simulink model "solar_thermal_sym"  (R2024b)
settings: Solver=FixedStepAuto  StartTime=0.0  StopTime=24*3600  FixedStep=60  RelTol=1e-3
values from neighbouring files (symbols this model uses):
  FR_consumption = 0*min    [Consumption_profiles.m]
  I_sym = I_feb    [Consumption_profiles.m]
  T_mains = 12    [Consumption_profiles.m]
  Ta_sym = Ta_feb    [Consumption_profiles.m]
  TR_consumption = 0*min    [Consumption_profiles.m]
undefined symbols (not defined in the file or in its folder): A, c, epsilon, eta_0, m_c, M_s, T_home, tank_LC, Tin_0, Ts_0, U
settings Model: Creator=edoardomurgia  LastModifiedBy=edoardomurgia
settings DataIOCC: ReturnWorkspaceOutputs=off
settings DebuggingCC: AlgebraicLoopMsg=none

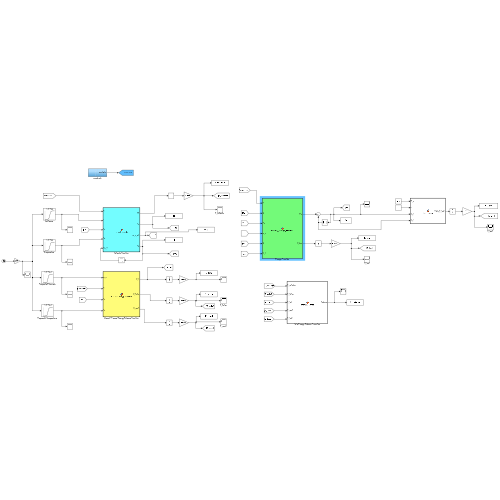
[thumbnail: Simulink's stored preview of the top-level diagram]
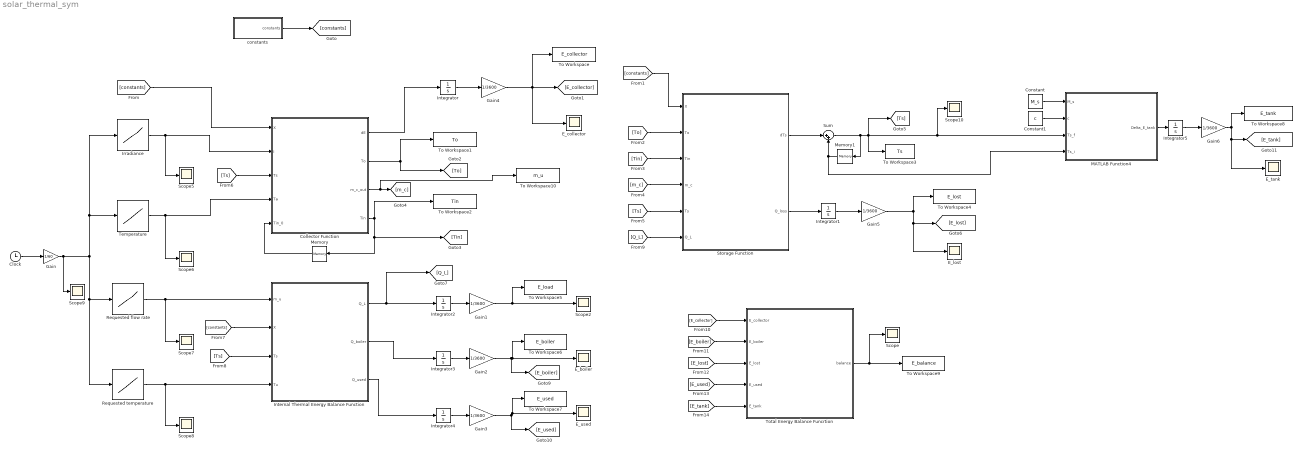
== system solar_thermal_sym ==
  Clock : Clock
  Collector Function : MATLAB Function  TreatAsAtomicUnit=on
  Constant : Constant  Value=M_s
  Constant1 : Constant  Value=c
  E_boiler : Scope
  E_collector : Scope
  E_lost : Scope
  E_tank : Scope
  E_used : Scope
  Gain : Gain  Gain=1/60
  Gain{1..6} (6 alike) : Gain  Gain=1/3600
  Integrator{,1..5} (6 alike) : Integrator
  Internal Thermal Energy Balance Function : MATLAB Function  TreatAsAtomicUnit=on
  Irradiance : Lookup_n-D  NumberOfTableDimensions=1  BreakpointsForDimension1=min  Table=I_sym  InternalRulePriority=Speed  RndMeth=Simplest
  MATLAB Function4 : MATLAB Function  TreatAsAtomicUnit=on
  Memory : Memory  InitialCondition=Tin_0
  Memory1 : Memory  InitialCondition=Ts_0
  Requested flow rate : Lookup_n-D  NumberOfTableDimensions=1  BreakpointsForDimension1=min  Table=FR_consumption  InternalRulePriority=Speed  RndMeth=Simplest
  Requested temperature : Lookup_n-D  NumberOfTableDimensions=1  BreakpointsForDimension1=min  Table=TR_consumption  InternalRulePriority=Speed  RndMeth=Simplest
  Scope{,2,5..10} (8 alike) : Scope
  Storage Function : MATLAB Function  TreatAsAtomicUnit=on
  Sum : Sum  Inputs=|++
  Temperature : Lookup_n-D  NumberOfTableDimensions=1  BreakpointsForDimension1=min  Table=Ta_sym  InternalRulePriority=Speed  RndMeth=Simplest
  To Workspace : ToWorkspace  VariableName=E_collector  SampleTime=-1
  To Workspace1 : ToWorkspace  VariableName=To  SampleTime=-1
  To Workspace10 : ToWorkspace  VariableName=m_u  SampleTime=-1
  To Workspace2 : ToWorkspace  VariableName=Tin  SampleTime=-1
  To Workspace3 : ToWorkspace  VariableName=Ts  SampleTime=-1
  To Workspace4 : ToWorkspace  VariableName=E_lost  SampleTime=-1
  To Workspace5 : ToWorkspace  VariableName=E_load  SampleTime=-1
  To Workspace6 : ToWorkspace  VariableName=E_boiler  SampleTime=-1
  To Workspace7 : ToWorkspace  VariableName=E_used  SampleTime=-1
  To Workspace8 : ToWorkspace  VariableName=E_tank  SampleTime=-1
  To Workspace9 : ToWorkspace  VariableName=E_balance  SampleTime=-1
  Total Energy Balance Funcrtion : MATLAB Function  TreatAsAtomicUnit=on
  constants : Subsystem
  wires:
  Clock/1 -> Gain/1
  constants/1(constants) -> [constants]
  [constants] -> Collector Function/1(X)
  Collector Function/4(Tin) -> Memory/1, [Tin], To Workspace2/1
  Memory/1 -> Collector Function/5(Tin_0)
  Collector Function/1(dE) -> Integrator/1
  Integrator/1 -> Gain4/1
  Collector Function/2(To) -> [To], To Workspace1/1
  [constants] -> Storage Function/1(X)
  [To] -> Storage Function/2(To)
  [Tin] -> Storage Function/3(Tin)
  [m_c] -> Storage Function/4(m_c)
  Storage Function/1(dTs) -> Sum/1
  [Ts] -> Storage Function/5(Ts)
  [Ts] -> Collector Function/3(Ts)
  Integrator1/1 -> Gain5/1
  Storage Function/2(Q_loss) -> Integrator1/1
  Gain/1 -> Requested temperature/1, Requested flow rate/1, Irradiance/1, Temperature/1, Scope9/1
  [constants] -> Internal Thermal Energy Balance Function/2(X)
  [Ts] -> Internal Thermal Energy Balance Function/3(Ts)
  [Q_L] -> Storage Function/6(Q_L)
  Internal Thermal Energy Balance Function/1(Q_L) -> Integrator2/1, [Q_L]
  Internal Thermal Energy Balance Function/2(Q_boiler) -> Integrator3/1
  Internal Thermal Energy Balance Function/3(Q_used) -> Integrator4/1
  [E_collector] -> Total Energy Balance Funcrtion/1(E_collector)
  [E_boiler] -> Total Energy Balance Funcrtion/2(E_boiler)
  Constant/1 -> MATLAB Function4/1(M_s)
  Memory1/1 -> MATLAB Function4/4(Ts_i), Sum/2
  MATLAB Function4/1(Delta_E_tank) -> Integrator5/1
  [E_tank] -> Total Energy Balance Funcrtion/5(E_tank)
  Total Energy Balance Funcrtion/1(balance) -> Scope/1, To Workspace9/1
  Integrator2/1 -> Gain1/1
  Integrator3/1 -> Gain2/1
  Integrator4/1 -> Gain3/1
  Irradiance/1 -> Scope5/1, Collector Function/2(I)
  Temperature/1 -> Scope6/1, Collector Function/4(Ta)
  Requested flow rate/1 -> Scope7/1, Internal Thermal Energy Balance Function/1(m_u)
  Requested temperature/1 -> Scope8/1, Internal Thermal Energy Balance Function/4(Tu)
  Sum/1 -> Memory1/1, MATLAB Function4/3(Ts_f), Scope10/1, To Workspace3/1, [Ts]
  Gain1/1 -> Scope2/1, To Workspace5/1
  Gain2/1 -> E_boiler/1, To Workspace6/1, [E_boiler]
  Gain4/1 -> E_collector/1, [E_collector], To Workspace/1
  Constant1/1 -> MATLAB Function4/2(c)
  Gain5/1 -> E_lost/1, [E_lost], To Workspace4/1
  Gain3/1 -> E_used/1, To Workspace7/1, [E_used]
  Collector Function/3(m_c_out) -> To Workspace10/1, [m_c]
  Gain6/1 -> E_tank/1, [E_tank], To Workspace8/1
  Integrator5/1 -> Gain6/1
  [E_lost] -> Total Energy Balance Funcrtion/3(E_lost)
  [E_used] -> Total Energy Balance Funcrtion/4(E_used)

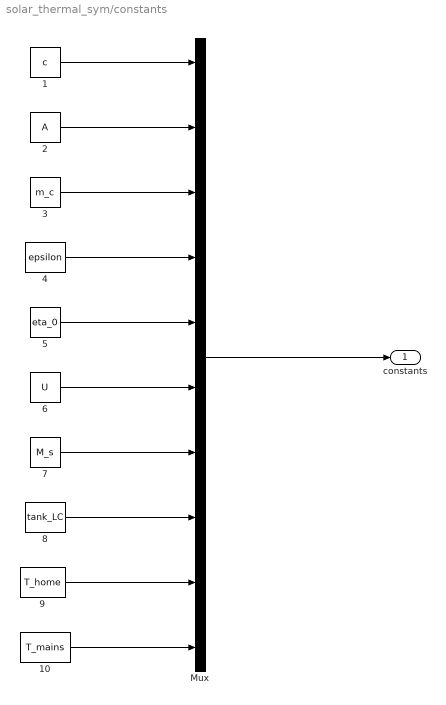
== system solar_thermal_sym/constants ==
  1 : Constant  Value=c
  10 : Constant  Value=T_mains
  2 : Constant  Value=A
  3 : Constant  Value=m_c
  4 : Constant  Value=epsilon
  5 : Constant  Value=eta_0
  6 : Constant  Value=U
  7 : Constant  Value=M_s
  8 : Constant  Value=tank_LC
  9 : Constant  Value=T_home
  Mux : Mux  Inputs=10
  constants : Outport
  wires:
  Mux/1 -> constants/1
  4/1 -> Mux/4
  8/1 -> Mux/8
  9/1 -> Mux/9
  7/1 -> Mux/7
  6/1 -> Mux/6
  5/1 -> Mux/5
  3/1 -> Mux/3
  2/1 -> Mux/2
  1/1 -> Mux/1
  10/1 -> Mux/10

== matlab function solar_thermal_sym/Storage Function ==
  data: X input; dTs output; To input; Tin input; m_c input; Ts input; Q_L input; Q_loss output
function [dTs,Q_loss] = thermal_storage_dynamics(X,To,Tin,m_c,Ts,Q_L)
    A       = X(2);
    c       = X(1);
    M_s      = X(7);
    tank_LC = X(8);
    T_home  = X(9);
    
    % Compute dTs using the given thermal energy balance equation:
    Q_loss = tank_LC*A*(Ts-T_home);
    
    dTs = (m_c * c * (To - Tin) - Q_L - Q_loss ) / (M_s * c);

end

== matlab function solar_thermal_sym/Collector Function ==
  data: X input; dE output; I input; Ts input; Ta input; Tin_0 input; To output; m_c_out output; Tin output
function [dE,To,m_c_out,Tin] = thermal_collector(X,I,Ts,Ta,Tin_0)

% Constants from MUX
c       = X(1);
A       = X(2);
m_c     = X(3);
epsilon = X(4);
eta_0   = X(5);
U       = X(6);


% Compute eta
if I <= 0
    eta = 0;
else
    eta = eta_0-U*(Tin_0-Ta)/I;
end

% If collector does not work
Tin = Ts;
To  = Ts;

% If collector is working compute  Tin and To
if (I > 0 && eta > 0)
    
    m_c_out = m_c;

    To = (eta*I*A)/(m_c*c*epsilon)+Ts;
    Tin = Ts+(eta*I*A)/(m_c*c)*(1/epsilon-1);

else
    m_c_out = 0;
end

dE = eta*I*A;

== matlab function solar_thermal_sym/Internal Thermal Energy Balance Function ==
  data: m_u input; X input; Ts input; Q_L output; Tu input; Q_boiler output; Q_used output
function [Q_L,Q_boiler,Q_used]  = thermal_energy_balance(m_u,X,Ts,Tu)
% MATLAB function to calculate heat losses and boiler contribution
    c  = X(1);
    Tm = X(10);
    
    % Compute Q_L (heat exchange with the storage tank)     4) On the notes
    if (Tu <= Ts)
        Q_L = m_u * c * (Tu - Tm);
    else
        Q_L = m_u * c * (Ts - Tm);
    end
    
    % Compute Q_boiler (boiler activation logic)            5) On the notes
    if (Tu <= Ts)
        Q_boiler = 0;                   % Boiler is not needed
    else
        Q_boiler = m_u * c * (Tu - Ts); % Boiler compensates thermal deficit
    end

    Q_used= m_u * c * (Tu - Tm);
end

== matlab function solar_thermal_sym/Total Energy Balance Funcrtion ==
  data: E_collector input; balance output; E_boiler input; E_lost input; E_used input; E_tank input
function balance = energy_balance(E_collector, E_boiler, E_lost, E_used, E_tank)

balance = E_collector + E_boiler - E_used - E_lost - E_tank;

== matlab function solar_thermal_sym/MATLAB Function4 ==
  data: M_s input; Delta_E_tank output; c input; Ts_f input; Ts_i input
function Delta_E_tank = delta_energy(M_s, c, Ts_f, Ts_i)

Delta_E_tank = M_s * c * (Ts_f-Ts_i);
